simulink model "aclarke_trans"  (R2015a)
settings: Solver=ode45  StartTime=0.0  StopTime=40/1000  RelTol=1e-3
settings Model: Creator=Windows 10  LastModifiedBy=Windows 10

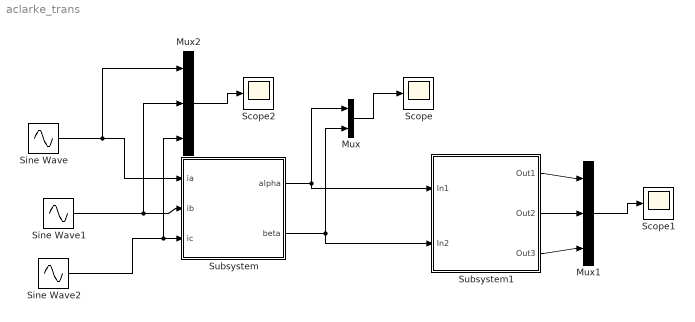
== system aclarke_trans ==
  Mux : Mux  Inputs=2
  Mux1 : Mux  Inputs=3
  Mux2 : Mux  Inputs=3
  Scope : Scope
  Scope1 : Scope
  Scope2 : Scope
      settings: SaveName=ScopeData2
  Sine Wave : Sin  Amplitude=180  Frequency=50*2*pi  SampleTime=0
  Sine Wave1 : Sin  Amplitude=180  Frequency=50*2*pi  Phase=-2*pi/3  SampleTime=0
  Sine Wave2 : Sin  Amplitude=180  Frequency=50*2*pi  Phase=2*pi/3  SampleTime=0
  Subsystem : Subsystem
  Subsystem1 : Subsystem
  wires:
  Mux1/1 -> Scope1/1
  Mux/1 -> Scope/1
  Subsystem/1(alpha) -> Mux/1, Subsystem1/1(In1)
  Subsystem/2(beta) -> Mux/2, Subsystem1/2(In2)
  Subsystem1/1(Out1) -> Mux1/1
  Subsystem1/3(Out3) -> Mux1/3
  Subsystem1/2(Out2) -> Mux1/2
  Mux2/1 -> Scope2/1
  Sine Wave/1 -> Mux2/1, Subsystem/1(ia)
  Sine Wave2/1 -> Mux2/3, Subsystem/3(ic)
  Sine Wave1/1 -> Mux2/2, Subsystem/2(ib)

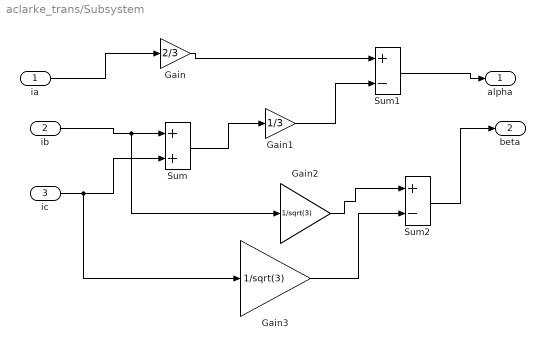
== system aclarke_trans/Subsystem ==
  ia : Inport
  ib : Inport  Port=2
  ic : Inport  Port=3
  Gain : Gain  Gain=2/3
  Gain1 : Gain  Gain=1/3
  Gain2 : Gain  Gain=1/sqrt(3)
  Gain3 : Gain  Gain=1/sqrt(3)
  Sum : Sum
  Sum1 : Sum  Inputs=+-
  Sum2 : Sum  Inputs=+-
  alpha : Outport
  beta : Outport  Port=2
  wires:
  Sum1/1 -> alpha/1
  Sum2/1 -> beta/1
  Gain/1 -> Sum1/1
  Gain1/1 -> Sum1/2
  Sum/1 -> Gain1/1
  ia/1 -> Gain/1
  ib/1 -> Gain2/1, Sum/1
  ic/1 -> Gain3/1, Sum/2
  Gain2/1 -> Sum2/1
  Gain3/1 -> Sum2/2

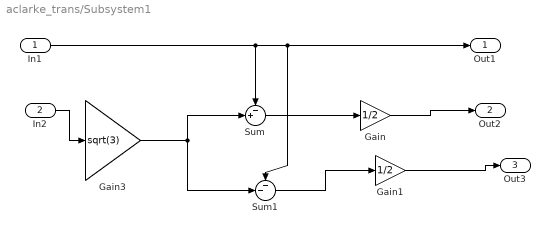
== system aclarke_trans/Subsystem1 ==
  In1 : Inport
  In2 : Inport  Port=2
  Gain : Gain  Gain=1/2
  Gain1 : Gain  Gain=1/2
  Gain3 : Gain  Gain=sqrt(3)
  Sum : Sum  Inputs=-+|
  Sum1 : Sum  Inputs=--|
  Out1 : Outport
  Out2 : Outport  Port=2
  Out3 : Outport  Port=3
  wires:
  Gain/1 -> Out2/1
  Gain1/1 -> Out3/1
  In2/1 -> Gain3/1
  Gain3/1 -> Sum/2, Sum1/2
  In1/1 -> Sum1/1, Out1/1, Sum/1
  Sum/1 -> Gain/1
  Sum1/1 -> Gain1/1
